simulink model "PT2_Param_limited Matlab"  (R2021a)
settings: Solver=ode45  StartTime=0.0  StopTime=10.0  FixedStep=1e-2  RelTol=1e-4  AbsTol=1e-4
values from neighbouring files (symbols this model uses):
  Kp = 9.8    [ITAE_Plots_PT2_limitations Rechenbeispiel.m]
  Tn = 4.7    [ITAE_Plots_PT2_limitations Rechenbeispiel.m]
  Tv = 0.3    [ITAE_Plots_PT2_limitations Rechenbeispiel.m]
settings Model: Creator=bhir  LastModifiedBy=bhir
settings SolverCC: AlgebraicLoopSolver=TrustRegion
settings DataIOCC: ReturnWorkspaceOutputs=off
settings DebuggingCC: SFMachineParentedDataDiag=warning  ArithmeticOperatorsInVariantConditions=warning
settings SFSimCC: SimUseLocalCustomCode=off  CustomCodeUndefinedFunction=UseInterfaceOnly
settings RTWCC: RTWUseLocalCustomCode=off
settings CodeAppCC: StateflowObjectComments=on

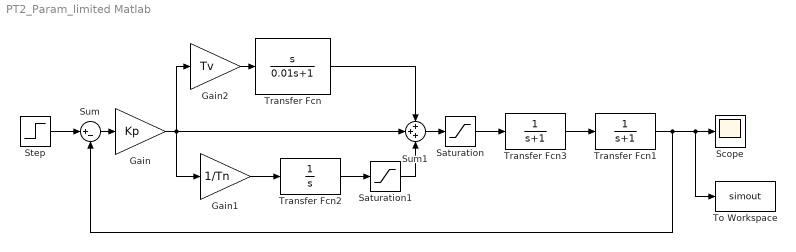
== system PT2_Param_limited Matlab ==
  Gain : Gain  Gain=Kp
  Gain1 : Gain  Gain=1/Tn
  Gain2 : Gain  Gain=Tv
  Saturation : Saturate  UpperLimit=5  LowerLimit=-5
  Saturation1 : Saturate  UpperLimit=5  LowerLimit=-5
  Scope : Scope
  Step : Step  Time=0  SampleTime=0
  Sum : Sum  Inputs=|+-
  Sum1 : Sum  Inputs=+++
  To Workspace : ToWorkspace  VariableName=simout  SaveFormat=Structure With Time  SampleTime=-1
  Transfer Fcn : TransferFcn  Numerator=[1 0]  Denominator=[0.01 1]
  Transfer Fcn1 : TransferFcn  Denominator=[1 1]
  Transfer Fcn2 : TransferFcn  Denominator=[1 0]
  Transfer Fcn3 : TransferFcn  Denominator=[1 1]
  wires:
  Step/1 -> Sum/1
  Sum/1 -> Gain/1
  Gain1/1 -> Transfer Fcn2/1
  Sum1/1 -> Saturation/1
  Gain/1 -> Gain2/1, Sum1/2, Gain1/1
  Transfer Fcn/1 -> Sum1/1
  Gain2/1 -> Transfer Fcn/1
  Transfer Fcn1/1 -> Sum/2, To Workspace/1, Scope/1
  Saturation/1 -> Transfer Fcn3/1
  Transfer Fcn3/1 -> Transfer Fcn1/1
  Transfer Fcn2/1 -> Saturation1/1
  Saturation1/1 -> Sum1/3
